simulink model "Stateflow_SDfixpoint2"  (R2015b)
settings: Solver=FixedStepDiscrete  StartTime=0.0  StopTime=10.0  RelTol=1e-3
settings Model: Creator=amyyang  LastModifiedBy=amyyang
settings OptimizationCC: DefaultParameterBehavior=Inlined  OptimizeModelRefInitCode=on  LifeSpan=1
settings DebuggingCC: SFUnusedDataAndEventsDiag=error
settings RTWCC: SystemTargetFile=ert.tlc  GenCodeOnly=on  TemplateMakefile=ert_default_tmf  Description=Embedded Coder  GenerateReport=on  IncludeHyperlinkInReport=on  LaunchReport=on  GenerateTraceInfo=on  GenerateTraceReport=on  GenerateTraceReportSl=on  GenerateTraceReportSf=on  GenerateTraceReportEml=on
settings CodeAppCC: IgnoreCustomStorageClasses=off
settings ERTTargetCC: GenerateSampleERTMain=on  InlinedParameterPlacement=NonHierarchical  ERTCustomFileTemplate=example_file_process.tlc

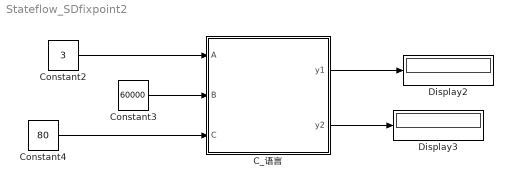
== system Stateflow_SDfixpoint2 ==
  C_语言 : Stateflow chart  TreatAsAtomicUnit=on
  Constant2 : Constant  Value=3  OutDataTypeStr=uint8
  Constant3 : Constant  Value=60000  OutDataTypeStr=uint16
  Constant4 : Constant  Value=80  OutDataTypeStr=fixdt(0,16,8)
  Display2 : Display
  Display3 : Display
  wires:
  Constant2/1 -> C_语言/1(A)
  Constant3/1 -> C_语言/2(B)
  C_语言/1(y1) -> Display2/1
  C_语言/2(y2) -> Display3/1
  Constant4/1 -> C_语言/3(C)

== stateflow chart Stateflow_SDfixpoint2/C_语言 ==
  (default) -> (junction 2) : {
      | // 冒号等于只能对单操作符起作用
      | y1 := ( A * B * C)/60000C;
      |
      | temp := A*B;
      | temp := temp*C;
      | y2 := temp/60000C;
      |
      | }
  data: A input; B input; C input; y1 output double; temp local double; y2 output double
